simulink model "controller_v4_2015a"  (R2015a)
settings: Solver=ode45  StartTime=0.0  StopTime=10.0  RelTol=1e-3
values from neighbouring files (symbols this model uses):
  De = 7.7*10^(-6)    (= 7.7e-06)    [WGS84_3D_UAS_User_Friendly.m]    (also in WGS84_3D_controller.m; WGS84_3D_controller_2015a.m; WGS84_3D_controller_FINAL.m; sim_3D_controller.m)
  gear = 0.001    [WGS84_3D_UAS_User_Friendly.m]    (also in WGS84_3D_controller.m; WGS84_3D_controller_2015a.m; WGS84_3D_controller_FINAL.m; sim_3D_controller.m)
  Je = 3*10^(-6)    (= 3e-06)    [WGS84_3D_UAS_User_Friendly.m]    (also in WGS84_3D_controller.m; WGS84_3D_controller_2015a.m; WGS84_3D_controller_FINAL.m; sim_3D_controller.m)
  Kb = 0.171    [WGS84_3D_UAS_User_Friendly.m]    (also in WGS84_3D_controller.m; WGS84_3D_controller_2015a.m; WGS84_3D_controller_FINAL.m; sim_3D_controller.m)
  Kt = 0.171    [WGS84_3D_UAS_User_Friendly.m]    (also in WGS84_3D_controller.m; WGS84_3D_controller_2015a.m; WGS84_3D_controller_FINAL.m; sim_3D_controller.m)
  La = 14.8*10^(-3)    (= 0.0148)    [WGS84_3D_UAS_User_Friendly.m]    (also in WGS84_3D_controller.m; WGS84_3D_controller_2015a.m; WGS84_3D_controller_FINAL.m; sim_3D_controller.m)
  lowSat = -5    [WGS84_3D_UAS_User_Friendly.m]    (also in WGS84_3D_controller.m; WGS84_3D_controller_2015a.m; WGS84_3D_controller_FINAL.m; sim_3D_controller.m)
  Ra = 25.6    [WGS84_3D_UAS_User_Friendly.m]    (also in WGS84_3D_controller.m; WGS84_3D_controller_2015a.m; WGS84_3D_controller_FINAL.m; sim_3D_controller.m)
  upSat = 5    [WGS84_3D_UAS_User_Friendly.m]    (also in WGS84_3D_controller.m; WGS84_3D_controller_2015a.m; WGS84_3D_controller_FINAL.m; sim_3D_controller.m)
libraries: simulink x8
settings Model: CovModelRefEnable=off  Creator=alvaro  LastModifiedBy=Orlando
settings DataIOCC: SaveFormat=Dataset
settings HardwareCC: ProdBitPerPointer=64  ProdLargestAtomicFloat=Float  ProdIntDivRoundTo=Zero  ProdEndianess=LittleEndian  ProdHWDeviceType=Specified
settings GRTTargetCC: GeneratePreprocessorConditionals=Use local settings

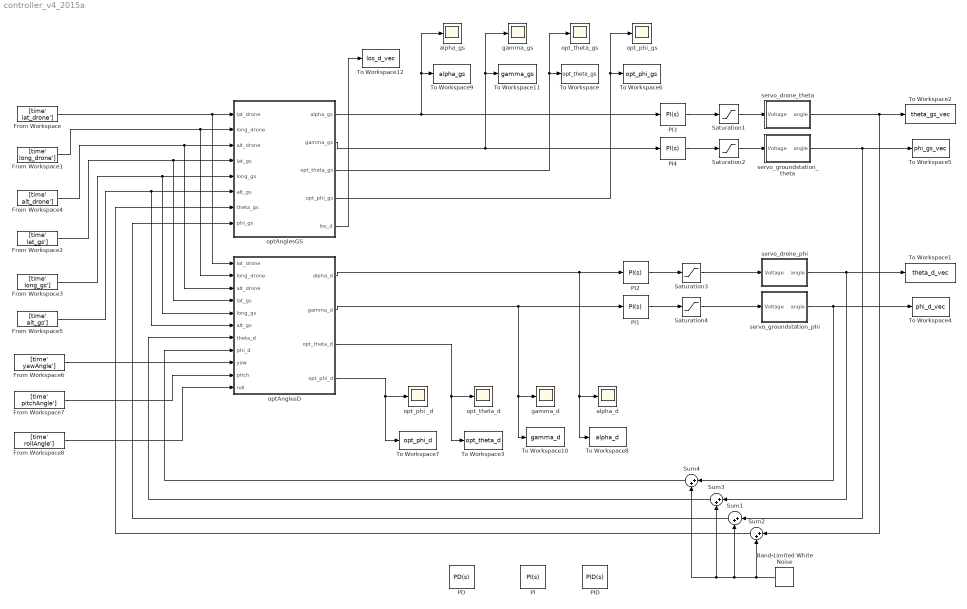
== system controller_v4_2015a ==
  Band-Limited White Noise : simulink/Sources/Band-Limited White Noise  Cov=[0.0001]  Ts=0.2  seed=[23341]
  From Workspace : FromWorkspace  VariableName=[time' lat_drone']  SampleTime=1
  From Workspace1 : FromWorkspace  VariableName=[time' long_drone']  OutDataTypeStr=double  SampleTime=1
  From Workspace2 : FromWorkspace  VariableName=[time' lat_gs']  SampleTime=1
  From Workspace3 : FromWorkspace  VariableName=[time' long_gs']  OutDataTypeStr=double  SampleTime=1
  From Workspace4 : FromWorkspace  VariableName=[time' alt_drone']  OutDataTypeStr=double  SampleTime=1
  From Workspace5 : FromWorkspace  VariableName=[time' alt_gs']  OutDataTypeStr=double  SampleTime=1
  From Workspace6 : FromWorkspace  VariableName=[time' yawAngle']  SampleTime=1
  From Workspace7 : FromWorkspace  VariableName=[time' pitchAngle']  SampleTime=1
  From Workspace8 : FromWorkspace  VariableName=[time' rollAngle']  SampleTime=1
  PD : simulink/Continuous/PID Controller  Controller=PD  TimeDomain=Continuous-time  SampleTime=-1  IntegratorMethod=Forward Euler  FilterMethod=Forward Euler  Form=Parallel  UseFilter=on  ControllerParametersSource=internal  P=7.39414726834109  I=0.0172882676140403  D=1.50790271020884  N=52.8940738192282  InitialConditionSource=internal  InitialConditionForIntegrator=0  InitialConditionForFilter=0  ExternalReset=none  LimitOutput=off  UpperSaturationLimit=inf  LowerSaturationLimit=-inf  LinearizeAsGain=on  AntiWindupMode=none  Kb=1  TrackingMode=off  Kt=1  PParamMin=[]  PParamMax=[]  IParamMin=[]  IParamMax=[]  DParamMin=[]  DParamMax=[]  NParamMin=[]  NParamMax=[]  KbParamMin=[]  KbParamMax=[]  KtParamMin=[]  KtParamMax=[]  POutMin=[]  POutMax=[]  IOutMin=[]  IOutMax=[]  DOutMin=[]  DOutMax=[]  NOutMin=[]  NOutMax=[]  KbOutMin=[]  KbOutMax=[]  KtOutMin=[]  KtOutMax=[]  IntegratorOutMin=[]  IntegratorOutMax=[]  FilterOutMin=[]  FilterOutMax=[]  SumOutMin=[]  SumOutMax=[]  SumI1OutMin=[]  SumI1OutMax=[]  SumI2OutMin=[]  SumI2OutMax=[]  SumI3OutMin=[]  SumI3OutMax=[]  SumDOutMin=[]  SumDOutMax=[]  SaturationOutMin=[]  SaturationOutMax=[]  IntegratorContinuousStateAttributes=''  IntegratorStateMustResolveToSignalObject=off  IntegratorRTWStateStorageClass=Auto  FilterContinuousStateAttributes=''  FilterStateMustResolveToSignalObject=off  FilterRTWStateStorageClass=Auto  DifferentiatorICPrevScaledInput=0  DifferentiatorOutMin=[]  DifferentiatorOutMax=[]
  PI{,1..4} (5 alike) : simulink/Continuous/PID Controller  Controller=PI  TimeDomain=Continuous-time  SampleTime=-1  IntegratorMethod=Forward Euler  FilterMethod=Forward Euler  Form=Parallel  UseFilter=on  ControllerParametersSource=internal  P=0.998635317234911  I=0.014417290883417  D=1.43723528432958  N=33.9607935997083  InitialConditionSource=internal  InitialConditionForIntegrator=0  InitialConditionForFilter=0  ExternalReset=none  LimitOutput=off  UpperSaturationLimit=inf  LowerSaturationLimit=-inf  LinearizeAsGain=on  AntiWindupMode=none  Kb=1  TrackingMode=off  Kt=1  PParamMin=[]  PParamMax=[]  IParamMin=[]  IParamMax=[]  DParamMin=[]  DParamMax=[]  NParamMin=[]  NParamMax=[]  KbParamMin=[]  KbParamMax=[]  KtParamMin=[]  KtParamMax=[]  POutMin=[]  POutMax=[]  IOutMin=[]  IOutMax=[]  DOutMin=[]  DOutMax=[]  NOutMin=[]  NOutMax=[]  KbOutMin=[]  KbOutMax=[]  KtOutMin=[]  KtOutMax=[]  IntegratorOutMin=[]  IntegratorOutMax=[]  FilterOutMin=[]  FilterOutMax=[]  SumOutMin=[]  SumOutMax=[]  SumI1OutMin=[]  SumI1OutMax=[]  SumI2OutMin=[]  SumI2OutMax=[]  SumI3OutMin=[]  SumI3OutMax=[]  SumDOutMin=[]  SumDOutMax=[]  SaturationOutMin=[]  SaturationOutMax=[]  IntegratorContinuousStateAttributes=''  IntegratorStateMustResolveToSignalObject=off  IntegratorRTWStateStorageClass=Auto  FilterContinuousStateAttributes=''  FilterStateMustResolveToSignalObject=off  FilterRTWStateStorageClass=Auto  DifferentiatorICPrevScaledInput=0  DifferentiatorOutMin=[]  DifferentiatorOutMax=[]
  PID : simulink/Continuous/PID Controller  Controller=PID  TimeDomain=Continuous-time  SampleTime=-1  IntegratorMethod=Forward Euler  FilterMethod=Forward Euler  Form=Parallel  UseFilter=on  ControllerParametersSource=internal  P=6.13715775557165  I=2.43593389565281  D=1.98468111231006  N=512.852311207883  InitialConditionSource=internal  InitialConditionForIntegrator=0  InitialConditionForFilter=0  ExternalReset=none  LimitOutput=off  UpperSaturationLimit=inf  LowerSaturationLimit=-inf  LinearizeAsGain=on  AntiWindupMode=none  Kb=1  TrackingMode=off  Kt=1  PParamMin=[]  PParamMax=[]  IParamMin=[]  IParamMax=[]  DParamMin=[]  DParamMax=[]  NParamMin=[]  NParamMax=[]  KbParamMin=[]  KbParamMax=[]  KtParamMin=[]  KtParamMax=[]  POutMin=[]  POutMax=[]  IOutMin=[]  IOutMax=[]  DOutMin=[]  DOutMax=[]  NOutMin=[]  NOutMax=[]  KbOutMin=[]  KbOutMax=[]  KtOutMin=[]  KtOutMax=[]  IntegratorOutMin=[]  IntegratorOutMax=[]  FilterOutMin=[]  FilterOutMax=[]  SumOutMin=[]  SumOutMax=[]  SumI1OutMin=[]  SumI1OutMax=[]  SumI2OutMin=[]  SumI2OutMax=[]  SumI3OutMin=[]  SumI3OutMax=[]  SumDOutMin=[]  SumDOutMax=[]  SaturationOutMin=[]  SaturationOutMax=[]  IntegratorContinuousStateAttributes=''  IntegratorStateMustResolveToSignalObject=off  IntegratorRTWStateStorageClass=Auto  FilterContinuousStateAttributes=''  FilterStateMustResolveToSignalObject=off  FilterRTWStateStorageClass=Auto  DifferentiatorICPrevScaledInput=0  DifferentiatorOutMin=[]  DifferentiatorOutMax=[]
  Saturation{1..4} (4 alike) : Saturate  UpperLimit=upSat  LowerLimit=lowSat
  Sum{1..4} (4 alike) : Sum  Inputs=|++
  To Workspace : ToWorkspace  VariableName=opt_theta_gs  SaveFormat=Timeseries  SampleTime=-1
  To Workspace1 : ToWorkspace  VariableName=theta_d_vec  SaveFormat=Timeseries  SampleTime=-1
  To Workspace10 : ToWorkspace  VariableName=gamma_d  SaveFormat=Timeseries  SampleTime=-1
  To Workspace11 : ToWorkspace  VariableName=gamma_gs  SaveFormat=Timeseries  SampleTime=-1
  To Workspace12 : ToWorkspace  VariableName=los_d_vec  SaveFormat=Timeseries  SampleTime=-1
  To Workspace2 : ToWorkspace  VariableName=theta_gs_vec  SaveFormat=Timeseries  SampleTime=-1
  To Workspace3 : ToWorkspace  VariableName=opt_theta_d  SaveFormat=Timeseries  SampleTime=-1
  To Workspace4 : ToWorkspace  VariableName=phi_d_vec  SaveFormat=Timeseries  SampleTime=-1
  To Workspace5 : ToWorkspace  VariableName=phi_gs_vec  SaveFormat=Timeseries  SampleTime=-1
  To Workspace6 : ToWorkspace  VariableName=opt_phi_gs  SaveFormat=Timeseries  SampleTime=-1
  To Workspace7 : ToWorkspace  VariableName=opt_phi_d  SaveFormat=Timeseries  SampleTime=-1
  To Workspace8 : ToWorkspace  VariableName=alpha_d  SaveFormat=Timeseries  SampleTime=-1
  To Workspace9 : ToWorkspace  VariableName=alpha_gs  SaveFormat=Timeseries  SampleTime=-1
  alpha_d : Scope
      settings: YMin=-10  YMax=10
  "alpha_gs " : Scope
      settings: YMin=-10  YMax=10  SaveName=ScopeData2
  gamma_d : Scope
      settings: YMin=-10  YMax=10  SaveName=ScopeData3
  gamma_gs : Scope
      settings: YMin=-10  YMax=10  SaveName=ScopeData4
  optAnglesD : MATLAB Function  TreatAsAtomicUnit=on
  "optAnglesGS " : MATLAB Function  TreatAsAtomicUnit=on
  opt_phi _d : Scope
      settings: YMin=-10  YMax=10  SaveName=ScopeData5
  opt_phi_gs : Scope
      settings: YMin=-10  YMax=10  SaveName=ScopeData6
  "opt_theta_d " : Scope
      settings: YMin=-10  YMax=10  SaveName=ScopeData7
  opt_theta_gs : Scope
      settings: YMin=-10  YMax=10
  servo_drone_phi : Subsystem
  servo_drone_theta : Subsystem
  servo_groundstation_phi : Subsystem
  servo_groundstation_theta : Subsystem
  wires:
  PI3/1 -> Saturation1/1
  PI4/1 -> Saturation2/1
  Saturation2/1 -> servo_groundstation_theta/1(Voltage)
  Saturation1/1 -> servo_drone_theta/1(Voltage)
  servo_groundstation_theta/1(angle) -> Sum1/1, To Workspace5/1
  PI2/1 -> Saturation3/1
  Saturation3/1 -> servo_drone_phi/1(Voltage)
  PI1/1 -> Saturation4/1
  Saturation4/1 -> servo_groundstation_phi/1(Voltage)
  servo_groundstation_phi/1(angle) -> To Workspace4/1, Sum4/1
  servo_drone_phi/1(angle) -> To Workspace1/1, Sum3/1
  servo_drone_theta/1(angle) -> Sum2/1, To Workspace2/1
  Band-Limited White Noise/1 -> Sum2/2, Sum4/2, Sum3/2, Sum1/2
  From Workspace/1 -> optAnglesD/1(lat_drone), "optAnglesGS "/1(lat_drone)
  From Workspace1/1 -> optAnglesD/2(long_drone), "optAnglesGS "/2(long_drone)
  From Workspace4/1 -> optAnglesD/3(alt_drone), "optAnglesGS "/3(alt_drone)
  From Workspace2/1 -> optAnglesD/4(lat_gs), "optAnglesGS "/4(lat_gs)
  From Workspace3/1 -> optAnglesD/5(long_gs), "optAnglesGS "/5(long_gs)
  From Workspace5/1 -> optAnglesD/6(alt_gs), "optAnglesGS "/6(alt_gs)
  Sum2/1 -> "optAnglesGS "/7(theta_gs)
  Sum1/1 -> "optAnglesGS "/8(phi_gs)
  Sum3/1 -> optAnglesD/7(theta_d)
  Sum4/1 -> optAnglesD/8(phi_d)
  "optAnglesGS "/1(alpha_gs) -> PI3/1, "alpha_gs "/1, To Workspace9/1
  "optAnglesGS "/2(gamma_gs) -> PI4/1, gamma_gs/1, To Workspace11/1
  "optAnglesGS "/3(opt_theta_gs) -> opt_theta_gs/1, To Workspace/1
  "optAnglesGS "/4(opt_phi_gs) -> opt_phi_gs/1, To Workspace6/1
  optAnglesD/1(alpha_d) -> PI2/1, alpha_d/1, To Workspace8/1
  optAnglesD/2(gamma_d) -> PI1/1, gamma_d/1, To Workspace10/1
  optAnglesD/3(opt_theta_d) -> "opt_theta_d "/1, To Workspace3/1
  optAnglesD/4(opt_phi_d) -> To Workspace7/1, opt_phi _d/1
  "optAnglesGS "/5(los_d) -> To Workspace12/1
  From Workspace6/1 -> optAnglesD/9(yaw)
  From Workspace7/1 -> optAnglesD/10(pitch)
  From Workspace8/1 -> optAnglesD/11(roll)

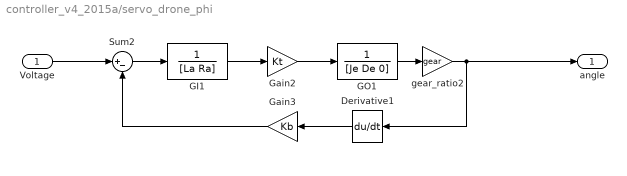
== system controller_v4_2015a/servo_drone_phi ==
  Voltage : Inport
  Derivative1 : Derivative
  GI1 : TransferFcn  Denominator=[La Ra]
  GO1 : TransferFcn  Denominator=[Je De 0]
  Gain2 : Gain  Gain=Kt
  Gain3 : Gain  Gain=Kb
  Sum2 : Sum  Inputs=|+-
  gear_ratio2 : Gain  Gain=gear
  angle : Outport
  wires:
  GI1/1 -> Gain2/1
  Gain2/1 -> GO1/1
  Derivative1/1 -> Gain3/1
  Gain3/1 -> Sum2/2
  Sum2/1 -> GI1/1
  Voltage/1 -> Sum2/1
  gear_ratio2/1 -> angle/1, Derivative1/1
  GO1/1 -> gear_ratio2/1

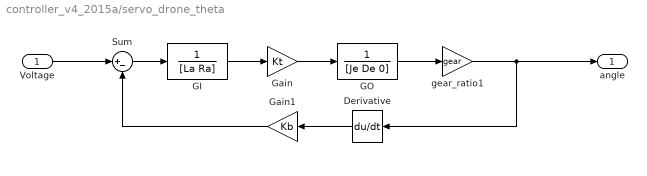
== system controller_v4_2015a/servo_drone_theta ==
  Voltage : Inport
  Derivative : Derivative
  GI : TransferFcn  Denominator=[La Ra]
  GO : TransferFcn  Denominator=[Je De 0]
  Gain : Gain  Gain=Kt
  Gain1 : Gain  Gain=Kb
  Sum : Sum  Inputs=|+-
  "gear_ratio1 " : Gain  Gain=gear
  angle : Outport
  wires:
  GO/1 -> "gear_ratio1 "/1
  Derivative/1 -> Gain1/1
  Sum/1 -> GI/1
  GI/1 -> Gain/1
  Gain1/1 -> Sum/2
  Gain/1 -> GO/1
  "gear_ratio1 "/1 -> angle/1, Derivative/1
  Voltage/1 -> Sum/1

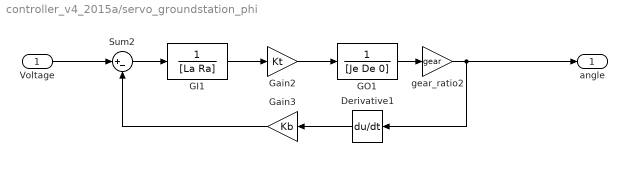
== system controller_v4_2015a/servo_groundstation_phi ==
  Voltage : Inport
  Derivative1 : Derivative
  GI1 : TransferFcn  Denominator=[La Ra]
  GO1 : TransferFcn  Denominator=[Je De 0]
  Gain2 : Gain  Gain=Kt
  Gain3 : Gain  Gain=Kb
  Sum2 : Sum  Inputs=|+-
  gear_ratio2 : Gain  Gain=gear
  angle : Outport
  wires:
  GI1/1 -> Gain2/1
  Gain2/1 -> GO1/1
  Derivative1/1 -> Gain3/1
  Gain3/1 -> Sum2/2
  Sum2/1 -> GI1/1
  Voltage/1 -> Sum2/1
  gear_ratio2/1 -> angle/1, Derivative1/1
  GO1/1 -> gear_ratio2/1

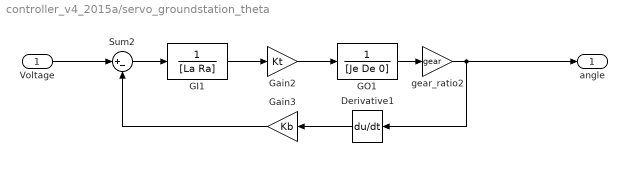
== system controller_v4_2015a/servo_groundstation_theta ==
  Voltage : Inport
  Derivative1 : Derivative
  GI1 : TransferFcn  Denominator=[La Ra]
  GO1 : TransferFcn  Denominator=[Je De 0]
  Gain2 : Gain  Gain=Kt
  Gain3 : Gain  Gain=Kb
  Sum2 : Sum  Inputs=|+-
  gear_ratio2 : Gain  Gain=gear
  angle : Outport
  wires:
  GI1/1 -> Gain2/1
  Gain2/1 -> GO1/1
  Derivative1/1 -> Gain3/1
  Gain3/1 -> Sum2/2
  Sum2/1 -> GI1/1
  Voltage/1 -> Sum2/1
  gear_ratio2/1 -> angle/1, Derivative1/1
  GO1/1 -> gear_ratio2/1

== matlab function controller_v4_2015a/optAnglesGS  ==
  data: lat_drone input; long_drone input; alt_drone input; lat_gs input; long_gs input; alt_gs input; theta_gs input; phi_gs input; alpha_gs output; gamma_gs output; opt_theta_gs output; opt_phi_gs output; los_d output
function [alpha_gs,gamma_gs,opt_theta_gs,opt_phi_gs,los_d] = ...
    optAnglesGS(lat_drone,long_drone,alt_drone,lat_gs,long_gs,alt_gs,theta_gs,phi_gs)
%**************************************************************************
%
% optAnglesGS.m - CA8 - DRONES
%
%**************************************************************************
%
% Group 832 - Control and Automation Msc.
% Aalborg University
% May 2016
%
%**************************************************************************
%
% DESCRIPTION:
% Function that performs the calculation for a 3 DIMENSION - 2 DEGREE OF
% FREEDOM 
%
% INPUTS:
% - x_drone = Position of the drone in X
% - y_drone = Position of the drone in Y
% - z_drone = Position of the drone in Z
% - x_gs = Position of the ground station in X
% - y_gs = Position of the ground station in Y
% - z_gs = Position of the ground station in Z
% - theta_gs = ANGLE of the ground station with respect to the X world
% - phi_gs = ANGLE of the ground station with respect to the Z world
%
% OUTPUTS:
% - alpha_gs = Angle from the direction of the pointing antenna of the ground station 
%   to the LINE OF SIGHT that joins ground station and drone. (SPHERICAL
%   COORDINATES)
% - phi_gs = Angle from the direction of the pointing antenna of the ground station 
%   to the LINE OF SIGHT that joins ground station and drone. (SPHERICAL
%   COORDINATES)
%
%**************************************************************************
%% Transform Drone position to Local NED GS

geoGS = [lat_gs;long_gs;alt_gs];
geoD = [lat_drone;long_drone;alt_drone];

ecefGS = geo2ecef(geoGS);
ecefD = geo2ecef(geoD);

nedD = ecef2ned(ecefD,geoGS);

x_drone = nedD(1);  % X = NORTH
y_drone = nedD(2);  % Y = EAST
z_drone = nedD(3);  % Z = DOWN

los_d = sqrt(x_drone^2 + y_drone^2 + z_drone^2);

% Optimal angle THETA
opt_theta_gs = atan2(x_drone,y_drone);

% Phi error calculations: GAMMA
opt_phi_gs = atan2(-z_drone,sqrt(abs(x_drone)^2 + abs(y_drone)^2));

% Error angles
alpha_gs = opt_theta_gs - theta_gs;
if (alpha_gs) > pi
    alpha_gs = -2*pi + alpha_gs;
elseif (alpha_gs) < -pi
    alpha_gs = 2*pi + alpha_gs;
end

gamma_gs = opt_phi_gs - phi_gs;
if (gamma_gs) > pi
    gamma_gs = -2*pi + gamma_gs;
elseif (alpha_gs) < -pi
    gamma_gs = 2*pi + gamma_gs;
end

end

== matlab function controller_v4_2015a/optAnglesD ==
  data: lat_drone input; long_drone input; alt_drone input; lat_gs input; long_gs input; alt_gs input; theta_d input; phi_d input; alpha_d output; gamma_d output; opt_theta_d output; opt_phi_d output; yaw input; pitch input; roll input
function [alpha_d,gamma_d,opt_theta_d,opt_phi_d] = ...
    optAnglesD(lat_drone,long_drone,alt_drone,lat_gs,long_gs,alt_gs,...
    theta_d,phi_d,yaw,pitch,roll)
%**************************************************************************
%
% optAnglesD.m - CA8 - DRONES
%
%**************************************************************************
%
% Group 832 - Control and Automation Msc.
% Aalborg University
% May 2016
%
%**************************************************************************
%
% DESCRIPTION:
%
% INPUTS:
%
% OUTPUTS:
%
%**************************************************************************
%% Transform Drone position to Local NED GS

geoGS = [lat_gs;long_gs;alt_gs];
geoD = [lat_drone;long_drone;alt_drone];

ecefGS = geo2ecef(geoGS);
ecefD = geo2ecef(geoD);

nedGS = ecef2ned(ecefGS,geoD);

bodyGS = ned2body(nedGS,yaw,pitch,roll);

x_gs = bodyGS(1);  % X = NORTH
y_gs = bodyGS(2);  % Y = EAST
z_gs = bodyGS(3);  % Z = DOWN

% Optimal angle THETA
opt_theta_d = atan2(x_gs,y_gs);

% Phi error calculations: GAMMA
opt_phi_d = atan2(-z_gs,sqrt(abs(x_gs)^2 + abs(y_gs)^2));

% Error angles
alpha_d = opt_theta_d - theta_d;
if (alpha_d) > pi
    alpha_d = -2*pi + alpha_d;
elseif (alpha_d) < -pi
    alpha_d = 2*pi + alpha_d;
end

gamma_d = opt_phi_d - phi_d;
if (gamma_d) > pi
    gamma_d = -2*pi + gamma_d;
elseif (gamma_d) < -pi
    gamma_d = 2*pi + gamma_d;
end

end
